simulink model "VB_IIR"  (R2020b)
settings: Solver=FixedStepDiscrete  StartTime=0.0  StopTime=Inf  RelTol=1e-3  EnableMultiTasking=on
libraries: dspsrcs4 x2, dspfdesign x1
settings Model: ModifiedByFormat=The MathWorks Inc.  Creator=The MathWorks, Inc.  LastModifiedBy=The MathWorks Inc.
settings DataIOCC: LimitDataPoints=on  SaveFormat=Array  SaveOutput=off  SignalLogging=off  DSMLogging=off  SaveTime=off  ReturnWorkspaceOutputs=off
settings OptimizationCC: DefaultParameterBehavior=Inlined  EnhancedBackFolding=on  PassReuseOutputArgsAs=Individual arguments  ZeroExternalMemoryAtStartup=off  ZeroInternalMemoryAtStartup=off  OptimizeBlockOrder=speed  DifferentSizesBufferReuse=on  OptimizationCustomize=off  EfficientTunableParamExpr=on
settings DebuggingCC: SolverPrmCheckMsg=warning  ParameterTunabilityLossMsg=error  AllowSymbolicDim=off  SFUnexpectedBacktrackingDiag=warning  SFNoUnconditionalDefaultTransitionDiag=warning  SFExecutionAtInitializationDiag=none  ArithmeticOperatorsInVariantConditions=warning
settings HardwareCC: ProdBitPerPointer=32  ProdBitPerSizeT=32  ProdBitPerPtrDiffT=32  ProdLargestAtomicFloat=None  ProdIntDivRoundTo=Undefined  ProdEndianess=Unspecified  ProdWordSize=32  ProdHWDeviceType=32-bit Generic
settings ModelReferenceCC: PropagateSignalLabelsOutOfModel=off
settings SFSimCC: SimUseLocalCustomCode=off  MATLABDynamicMemAlloc=off  CustomCodeUndefinedFunction=UseInterfaceOnly
settings RTWCC: Description=Embedded Coder  SystemTargetFile=ert.tlc  GenCodeOnly=on  TemplateMakefile=ert_default_tmf  RTWUseLocalCustomCode=off
settings CodeAppCC: ForceParamTrailComments=on  IgnoreCustomStorageClasses=off  OperatorAnnotations=on  SimulinkDataObjDesc=on  SFDataObjDesc=on  InsertBlockDesc=on
settings ERTTargetCC: GenerateSampleERTMain=on  InlinedParameterPlacement=NonHierarchical  ERTCustomFileTemplate=example_file_process.tlc
settings ConfigComp: CovMetricSettings=dw  CovSaveCumulativeToWorkspaceVar=on  CovSaveSingleToWorkspaceVar=on  CovExternalEMLEnable=off  CovSFcnEnable=off

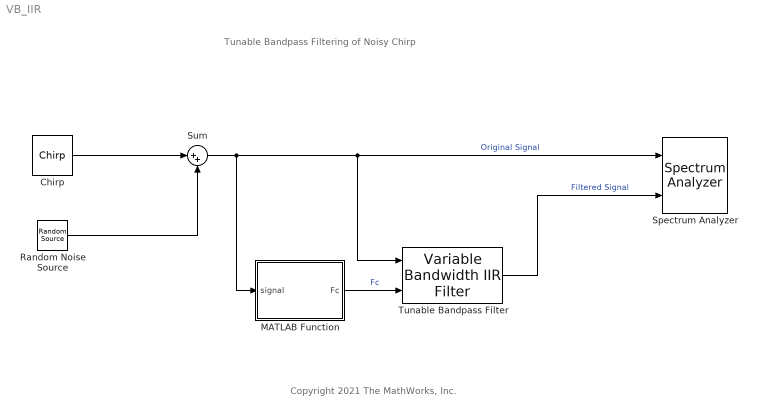
== system VB_IIR ==
  note: Tunable Bandpass Filtering of Noisy Chirp
  note: Copyright 2021 The MathWorks, Inc.
  Chirp : dspsrcs4/Chirp  sweep=Linear  mode=Bidirectional  f0=5000  f1=8000  t1=30  Tsweep=30  phase=0  Ts=1/44100  spf=1024  datatype=Double  OutputFrames=off
      settings: SourceProductName=DSP System Toolbox
  MATLAB Function : MATLAB Function  TreatAsAtomicUnit=on
  Random Noise Source : dspsrcs4/Random Source  SrcType=Gaussian  NormMethod=Ziggurat  CltLength=12  MinVal=0  MaxVal=1  MeanVal=0  VarVal=1e-5  RepMode=Specify seed  rawSeed=3  IsInherit=off  SampMode=Discrete  SampTime=1/44100  SampFrame=1024  DataType=Double  OutComplex=Real  OutputFrames=off
  Spectrum Analyzer : SpectrumAnalyzer  NumInputPorts=2
  Sum : Sum  Inputs=|++
  Tunable Bandpass Filter : dspfdesign/Variable Bandwidth IIR Filter  FilterType=Bandpass  FilterOrder=8  PassbandFrequencyPort=off  PassbandFrequency=7000  CenterFrequencyPort=on  CenterFrequency=10000  BandwidthPort=off  Bandwidth=1250  PassbandRipple=1  StopbandAttenuation=60  InheritSampleRate=off  SampleRate=44100  SimulateUsing=Interpreted execution
      settings: SourceProductName=DSP System Toolbox
  wires:
  Sum/1 -> Tunable Bandpass Filter/1, Spectrum Analyzer/1, MATLAB Function/1(signal)  "Original Signal"
  Chirp/1 -> Sum/1
  Random Noise Source/1 -> Sum/2
  Tunable Bandpass Filter/1 -> Spectrum Analyzer/2  "Filtered Signal"
  MATLAB Function/1(Fc) -> Tunable Bandpass Filter/2  "Fc"

== matlab function VB_IIR/MATLAB Function ==
  data: signal input; Fc output double size=1
% Copyright 2021 The MathWorks, Inc.

function Fc = CenterFreq(signal)
    Fs = 44100; % Sampling Rate of original signal (Hz)
 
    [pxx, f] = pwelch(signal,500,300,500,Fs); % Obtain Welch's overlapped segment averaging PSD
                                              % estimate of the signal
    [~,idx] = max(pxx);
    
    temp = f(idx);
    
    Fc = temp(1);
